simulink model "EKF_only"  (R2018b)
settings: Solver=ode4  StartTime=0.0  StopTime=300  FixedStep=0.06  MaxStep=0.1  RelTol=1e-3  AbsTol=1e-6
StartFcn:
  | clear radarLogsOut
StopFcn:
  | aero_radplot;
model workspace (MATLAB code in the model file):
  | dt = 0.02;  % Radar update rate (also hard-coded in extkalman.m)
CloseFcn:
  | h=findobj('type','figure');if ~isempty(h);close(h);end
  | clear radarLogsOut
Description:
  | Radar Tracking Using MATLAB(R) Function Block
  | 
  | This example shows how to use an extended Kalman filter with the
  | MATLAB(R) Function block in Simulink(R) to estimate an aircraft's
  | position from radar measurements. The filter implementation is found in the
  | MATLAB Function block, the contents of which are stored in the
  | Simulink model itself.
  | 
  | At the end of the simulation, three figures display the following information: the
  | actual trajectory compared to the estimated trajectory; the estimation residual
  | for range; and the actual, measured, and estimated positions.
settings Model: ExtModeTrigMode=oneshot  ExtModeArmWhenConnect=off  ExtModeAutoUpdateStatusClock=off  Creator=The MathWorks Inc.  LastModifiedBy=user
settings SolverCC: AutoScaleAbsTol=off
settings DataIOCC: SaveFormat=Array  SaveOutput=off  SaveTime=off  TimeSaveName=t_sim  SignalLoggingName=radarLogsOut
settings OptimizationCC: DefaultParameterBehavior=Inlined  InlineInvariantSignals=on  ExpressionDepthLimit=2147483647  StateBitsets=on  DataBitsets=on  ZeroExternalMemoryAtStartup=off  ZeroInternalMemoryAtStartup=off  NoFixptDivByZeroProtection=on  LifeSpan=1  BufferReusableBoundary=off
settings DebuggingCC: SaveWithParameterizedLinksMsg=none  UnderspecifiedInitializationDetection=Classic  MergeDetectMultiDrivingBlocksExec=none  CheckExecutionContextPreStartOutputMsg=on  CheckExecutionContextRuntimeOutputMsg=on  SignalResolutionControl=TryResolveAllWithWarning  MultiTaskDSMMsg=warning  MultiTaskCondExecSysMsg=none  FcnCallInpInsideContextMsg=warning  StateNameClashWarn=warning  SFUnexpectedBacktrackingDiag=warning  SFNoUnconditionalDefaultTransitionDiag=warning  SFExecutionAtInitializationDiag=none
settings HardwareCC: ProdBitPerPointer=32  ProdBitPerSizeT=32  ProdBitPerPtrDiffT=32  ProdLargestAtomicFloat=None  ProdIntDivRoundTo=Undefined  ProdEndianess=Unspecified  ProdWordSize=32  ProdHWDeviceType=32-bit Generic
settings ModelReferenceCC: PropagateSignalLabelsOutOfModel=off
settings SFSimCC: SimUseLocalCustomCode=off  SimParseCustomCode=off  MATLABDynamicMemAlloc=off
settings RTWCC: SystemTargetFile=ert.tlc  TLCOptions=-p0 -aWarnNonSaturatedBlocks=0  TemplateMakefile=ert_default_tmf  Description=RTW Embedded Coder (no auto configuration)  GenerateReport=on  RTWVerbose=off  RTWUseLocalCustomCode=off  IncludeHyperlinkInReport=on  LaunchReport=on
settings CodeAppCC: ForceParamTrailComments=on  IgnoreCustomStorageClasses=off  SimulinkDataObjDesc=on  CustomSymbolStrType=$N$R$M  CustomSymbolStrFcn=$F$N$M  CustomSymbolStrMacro=$N$M  InsertBlockDesc=on  StateflowObjectComments=on  InternalIdentifier=Classic
settings ERTTargetCC: TargetFcnLib=ansi_tfl_tmw.mat  MultiwordLength=2048  GenerateSampleERTMain=on  IncludeMdlTerminateFcn=off  SupportComplex=off  SupportContinuousTime=on  SupportNonInlinedSFcns=on  InlinedParameterPlacement=NonHierarchical  ERTCustomFileTemplate=example_file_process.tlc  ConvertIfToSwitch=off  SuppressUnreachableDefaultCases=off
settings ConfigComp: CovMetricSettings=d  CovHtmlReporting=on  CovSaveCumulativeToWorkspaceVar=on  CovSaveSingleToWorkspaceVar=on  CovExternalEMLEnable=off

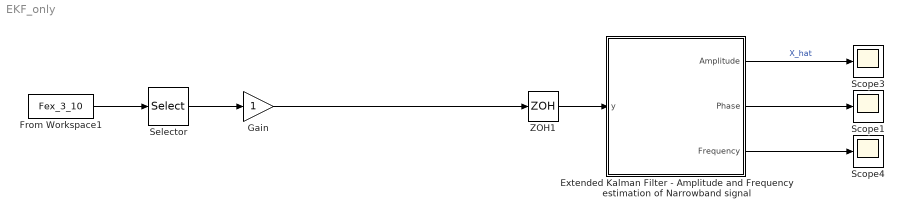
== system EKF_only ==
  Extended Kalman Filter - Amplitude and Frequency estimation of Narrowband signal : MATLAB Function  TreatAsAtomicUnit=on
  From Workspace1 : FromWorkspace  VariableName=Fex_3_10  SampleTime=0
  Gain : Gain
  Scope1 : Scope
  Scope3 : Scope
  Scope4 : Scope
  Selector : Selector  InputPortWidth=6  IndexOptions=Index vector (dialog)  Indices=1  OutputSizes=1
  ZOH1 : ZeroOrderHold  SampleTime=0.06
  wires:
  ZOH1/1 -> Extended Kalman Filter - Amplitude and Frequency estimation of Narrowband signal/1(y)
  Extended Kalman Filter - Amplitude and Frequency estimation of Narrowband signal/1(Amplitude) -> Scope3/1  "X_hat"
  Extended Kalman Filter - Amplitude and Frequency estimation of Narrowband signal/2(Phase) -> Scope1/1
  Extended Kalman Filter - Amplitude and Frequency estimation of Narrowband signal/3(Frequency) -> Scope4/1
  From Workspace1/1 -> Selector/1
  Selector/1 -> Gain/1
  Gain/1 -> ZOH1/1

== matlab function EKF_only/Extended Kalman Filter - Amplitude and Frequency estimation of Narrowband signal ==
  data: y input; Amplitude output double; Phase output; Frequency output
function [Amplitude, Phase, Frequency]   = EKF_narrowband(y)

% Initialization
persistent P;
persistent x;

dt = 0.06; %edit this to match your timestep

if isempty(P)
    x = [0 0 0.1]';       %state estimate
    P = diag([1e0 1e0 1e0]);    %Covariance matrix
end

%%%%%%%%%%%From Fusco thesis%%%%%%%%%%%%%%%%%%%%%
%%%State vector X = [a theta w]
x1 = x(1);  %Amplitude
x2 = x(2);  %Phase
w = x(3);   %frequency

%State transition matrices
A = [cos(w*dt) sin(w*dt) 0;
    -sin(w*dt) cos(w*dt) 0;
    0 0 1];

q1 = 1e11; q2 = 1e-1; q3 = 1e-2;%Must be comparable to expected magnitudes of each state

% q = [rand*q1 rand*q2 rand*q3]';
% Q = diag(q);
% R=rand*0.1;

q = [q1 q2 q3]';
Q = diag(q);
R=1e-1; %Measurement noise

%Jacobian
dA = [cos(w*dt) sin(w*dt) (-dt*x1*sin(w*dt) + dt*x2*cos(w*dt));
    -sin(w*dt) cos(w*dt) (-dt*x1*cos(w*dt) - dt*x2*sin(w*dt));
     0 0 1];
F = [(x1*cos(w*dt) + x2*sin(w*dt)); (-x1*sin(w*dt) + x2*cos(w*dt)); w];
C = [1 0 0];

%EKF predict/correct
x = A*x;
P = dA*P*dA' + Q;

S = C*P*C' + R;
K = P*C'/S;
x = x + K*(y-C*x);
P = (eye(3) - K*C)*P;

%outputs
Amplitude = sqrt(x(1)^2 + x(2)^2);
Frequency = x(3);
Phase = x(2);
